simulink model "heli_master_2015b"  (R2015b)
settings: Solver=ode1  SolverMode=SingleTasking  StartTime=0.0  StopTime=inf  FixedStep=0.002  RelTol=1e-3
PostLoadFcn:
  | qc_set_target_type(getConfigSet(bdroot, 'QUARC Default Target Configuration'));
values from neighbouring files (symbols this model uses):
  K = P_predicted * C' * inv(C * P_predicted * C' + obj.W)    [ExtendedKalmanFilter.m]    (also in HighGainObserver.m = zeros(8, 2); StateFeedback.m = zeros(2, 6))
  lamb = block.ContStates.Data(3)    [BetterSimulation.m]    (also in FeedbackLinearization.m = x(3); dyn_ext_eps_meas.mat = [0 0 0 0 0 0 0 0 0 0 0 0 ... (30000 elements, 6000x5)]; e_-10_10_l_0_120_t_10.mat = [0 3.40359280049e-12 1.08295188827e-10 8.177826625e-10 3.426; e_-10_10_l_0_120_t_20.mat = [0 1.06295178385e-13 3.38915391498e-12 2.56636695446e-11 1.0)
  phi = block.ContStates.Data(1)    [BetterSimulation.m]    (also in FeedbackLinearization.m = x(1); dyn_ext_eps_meas.mat = [0 0 0 0 0 0 0 0 0 0 0 0 ... (18000 elements, 6000x3)]; e_-10_10_l_0_120_t_10.mat = [3.57789727367e-14 3.32260230971e-07 2.63920782562e-06 8.843; e_-10_10_l_0_120_t_20.mat = [3.52494450884e-15 1.04005854531e-08 8.29611824462e-08 2.791)
  R = diag(R_diag)    [compute_lqr_feedback.m]    (also in first_tvlqr_test.mat = [1  0; 0  1])
  vb = block.InputPort(2).Data    [BetterSimulation.m]    (also in analyze_eps_meas.m = [log_neg.signals(2).values; log_pos.signals(2).values]; dyn_ext_eps_meas.mat = [2.46662433384 2.46662437608 2.46662467016 2.46662546356 2.4; e_-10_10_l_0_120_t_10.mat = [3.03305943788 3.0306076999 3.02819113358 3.02581096907 3.02; e_-10_10_l_0_120_t_20.mat = [3.03305943788 3.0329822422 3.03290486178 3.03282733913 3.03)
  vf = block.InputPort(1).Data    [BetterSimulation.m]    (also in analyze_eps_meas.m = [log_neg.signals(1).values; log_pos.signals(1).values]; dyn_ext_eps_meas.mat = [2.46662433384 2.46662437608 2.46662467016 2.46662546356 2.4; e_-10_10_l_0_120_t_10.mat = [3.03305943788 3.03551133878 3.03792903521 3.04031223633 3.0; e_-10_10_l_0_120_t_20.mat = [3.03305943788 3.03313663866 3.03321405463 3.03329167331 3.0)
undefined symbols (not defined in the file or in its folder): HIL, qc_get_step_size
libraries: simulink_extras x25, quarc_library x4
(part 2 of 2)

== system heli_master_2015b/Feedback Controller/Trajectory Controller/Enabled Controller/Trajectory Controller Variants/TimeVariantLQR ==
  t : Inport
  x : Inport  Port=2
  t_d : Inport  Port=3
  phi_d : Inport  Port=4
  eps_d : Inport  Port=5
  lamb_d : Inport  Port=6
  vf_d : Inport  Port=7
  vb_d : Inport  Port=8
  MATLAB System : MATLABSystem  System=TimeVariantLQR  Q=Q  R=R  S=S  riccati_tau=riccati_tau  riccati_P_triu_tau=riccati_P_triu_tau  SimulateUsing=Code generation
      mask Type: TimeVariantLQR
      mask Display:
      | disp('TimeVariantLQR');
      | port_label('input',1,'Time');
      | port_label('input',2,'State');
      | port_label('input',3,'Traj Time');
      | port_label('input',4,'Traj Phi');
      | port_label('input',5,'Traj Eps');
      | port_label('input',6,'Traj Lamb');
      | port_label('input',7,'Traj Vf');
      | port_label('input',8,'Traj Vb');
      | port_label('output',1,'Control');
  TimeVariantLQR : Subsystem  Commented=on  mask(Time Variant LQR){Q_diag=[3, 50, 20, 2, 1, 5, 1, 1], R_diag=[1, 1], S_diag=[3, 50, 20, 2, 1, 5, 1, 1], riccati_step_width=0.1}
      mask help: LQR for LTV system resulting from linearization around desired trajectory.
      mask DialogControl Control2 Prompt: diag(Q):
      mask DialogControl Control3 Prompt: diag(R):
      mask DialogControl Control3_copy Prompt: diag(S):
      mask DialogControl Control4 Prompt: Riccati step width:
  u : Outport
  wires:
  MATLAB System/1 -> u/1
  vb_d/1 -> MATLAB System/8
  vf_d/1 -> MATLAB System/7
  lamb_d/1 -> MATLAB System/6
  eps_d/1 -> MATLAB System/5
  phi_d/1 -> MATLAB System/4
  t_d/1 -> MATLAB System/3
  x/1 -> MATLAB System/2
  t/1 -> MATLAB System/1

== system heli_master_2015b/Feedback Controller/Trajectory Controller/Enabled Controller/Trajectory Controller Variants/TimeVariantLQRI ==
  t : Inport
  x : Inport  Port=2
  t_d : Inport  Port=3
  phi_d : Inport  Port=4
  eps_d : Inport  Port=5
  lamb_d : Inport  Port=6
  vf_d : Inport  Port=7
  vb_d : Inport  Port=8
  MATLAB System : MATLABSystem  System=TimeVariantLQRI  Q=Q  R=R  S=S  riccati_tau=riccati_tau  riccati_P_triu_tau=riccati_P_triu_tau  step_width=0.002  SimulateUsing=Code generation
      mask Type: TimeVariantLQRI
      mask Display:
      | disp('TimeVariantLQRI');
      | port_label('input',1,'Time');
      | port_label('input',2,'State');
      | port_label('input',3,'Traj Time');
      | port_label('input',4,'Traj Phi');
      | port_label('input',5,'Traj Eps');
      | port_label('input',6,'Traj Lamb');
      | port_label('input',7,'Traj Vf');
      | port_label('input',8,'Traj Vb');
      | port_label('output',1,'Control');
      | port_label('output',2,'Debug');
  u : Outport
  wires:
  MATLAB System/1 -> u/1
  vb_d/1 -> MATLAB System/8
  vf_d/1 -> MATLAB System/7
  lamb_d/1 -> MATLAB System/6
  eps_d/1 -> MATLAB System/5
  phi_d/1 -> MATLAB System/4
  t_d/1 -> MATLAB System/3
  x/1 -> MATLAB System/2
  t/1 -> MATLAB System/1

== system heli_master_2015b/Feedback Controller/Trajectory Controller/Enabled Controller/Trajectory Controller Variants/Ad hoc PID/Conversion ==
  Vd [V] : Inport
  Vs [V] : Inport  Port=2
  Add : Sum
  Back gain : Gain  Gain=0.5
  Front gain : Gain  Gain=0.5
  Subtract : Sum  Inputs=+-
  Vf [V] : Outport
  Vb [V] : Outport  Port=2
  wires:
  Vd [V]/1 -> Subtract/2, Add/1
  Vs [V]/1 -> Subtract/1, Add/2
  Subtract/1 -> Back gain/1
  Back gain/1 -> Vb [V]/1
  Add/1 -> Front gain/1
  Front gain/1 -> Vf [V]/1

== system heli_master_2015b/Feedback Controller/Trajectory Controller/Enabled Controller/Trajectory Controller Variants/Ad hoc PID/Elevation controller ==
  e~ [rad] : Inport
  e~dot [rad/s] : Inport  Port=2
  e~c [rad] : Inport  Port=3
  Elevation controller : Subsystem
  Sum : Sum  Inputs=-+  SaturateOnIntegerOverflow=on  InputSameDT=on  OutDataTypeStr=Inherit: Same as first input
  V~s [V] : Outport  InitialOutput=0
  wires:
  Sum/1 -> Elevation controller/1(e~ [rad])
  Elevation controller/1(V~_s [V]) -> V~s [V]/1
  e~ [rad]/1 -> Sum/1
  e~dot [rad/s]/1 -> Elevation controller/2(e~_dot [rad/s])
  e~c [rad]/1 -> Sum/2

== system heli_master_2015b/Feedback Controller/Trajectory Controller/Enabled Controller/Trajectory Controller Variants/Ad hoc PID/Pitch controller ==
  p~c [rad] : Inport
  p~ [rad] : Inport  Port=2
  p~dot [rad/s] : Inport  Port=3
  Integrator : Integrator  LimitOutput=on
  Kd : Gain  Gain=3.5
  Ki : Gain  Gain=0.5
  Kp : Gain  Gain=8
  Saturation : Saturate  UpperLimit=10  LowerLimit=-10
  Sum : Sum  Inputs=+-
  Sum1 : Sum  Inputs=++-
  V~d [V] : Outport  InitialOutput=0
  wires:
  p~c [rad]/1 -> Sum/1
  p~ [rad]/1 -> Sum/2
  Sum/1 -> Ki/1, Kp/1
  p~dot [rad/s]/1 -> Kd/1
  Kp/1 -> Sum1/1
  Sum1/1 -> Saturation/1
  Saturation/1 -> V~d [V]/1
  Kd/1 -> Sum1/3
  Ki/1 -> Integrator/1
  Integrator/1 -> Sum1/2

== system heli_master_2015b/Feedback Controller/Trajectory Controller/Enabled Controller/Trajectory Controller Variants/Ad hoc PID/Travel controller ==
  lamb~c [rad] : Inport
  lamb~ [rad] : Inport  Port=2
  lamb~dot [rad/s] : Inport  Port=3
  Integrator : Integrator  LimitOutput=on  UpperSaturationLimit=45/180*pi  LowerSaturationLimit=-45/180*pi
  Kd : Gain  Gain=1.2
  Ki : Gain  Gain=0.02
  Kp : Gain  Gain=0.7
  Saturation : Saturate  UpperLimit=45/180*pi  LowerLimit=-45/180*pi
  Sum : Sum  Inputs=+-
  Sum1 : Sum  Inputs=++-
  p~c [rad] : Outport  InitialOutput=0
  wires:
  lamb~c [rad]/1 -> Sum/1
  lamb~ [rad]/1 -> Sum/2
  Sum/1 -> Ki/1, Kp/1
  lamb~dot [rad/s]/1 -> Kd/1
  Kp/1 -> Sum1/1
  Saturation/1 -> p~c [rad]/1
  Kd/1 -> Sum1/3
  Ki/1 -> Integrator/1
  Integrator/1 -> Sum1/2
  Sum1/1 -> Saturation/1

== system heli_master_2015b/Feedback Controller/Trajectory Controller/Enabled Controller/Trajectory Controller Variants/Joystick PID/Conversion ==
  Vd [V] : Inport
  Vs [V] : Inport  Port=2
  Add : Sum
  Back gain : Gain  Gain=0.5
  Front gain : Gain  Gain=0.5
  Subtract : Sum  Inputs=+-
  Vf [V] : Outport
  Vb [V] : Outport  Port=2
  wires:
  Vd [V]/1 -> Subtract/2, Add/1
  Vs [V]/1 -> Subtract/1, Add/2
  Subtract/1 -> Back gain/1
  Back gain/1 -> Vb [V]/1
  Add/1 -> Front gain/1
  Front gain/1 -> Vf [V]/1

== system heli_master_2015b/Feedback Controller/Trajectory Controller/Enabled Controller/Trajectory Controller Variants/Joystick PID/Elevation controller ==
  e~ [rad] : Inport
  e~dot [rad/s] : Inport  Port=2
  e~c [rad] : Inport  Port=3
  Elevation controller : Subsystem
  Sum : Sum  Inputs=-+  SaturateOnIntegerOverflow=on  InputSameDT=on  OutDataTypeStr=Inherit: Same as first input
  V~s [V] : Outport  InitialOutput=0
  wires:
  Sum/1 -> Elevation controller/1(e~ [rad])
  Elevation controller/1(V~_s [V]) -> V~s [V]/1
  e~ [rad]/1 -> Sum/1
  e~dot [rad/s]/1 -> Elevation controller/2(e~_dot [rad/s])
  e~c [rad]/1 -> Sum/2

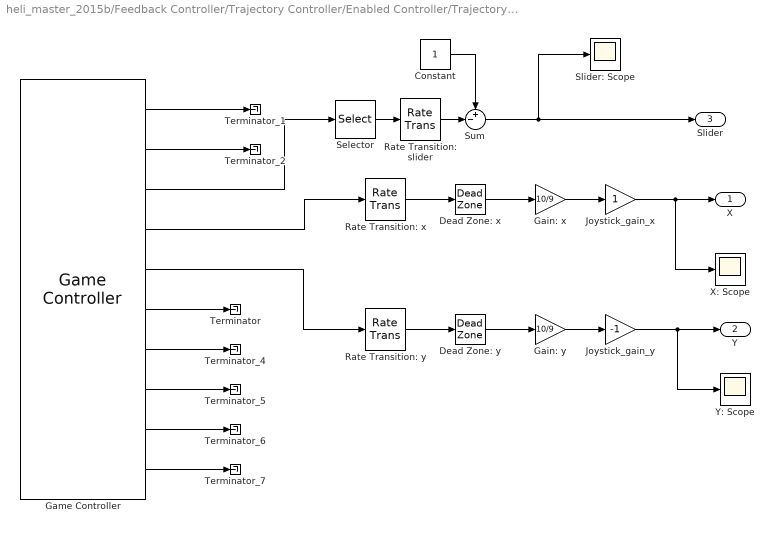
== system heli_master_2015b/Feedback Controller/Trajectory Controller/Enabled Controller/Trajectory Controller Variants/Joystick PID/Joystick ==
  Constant : Constant
  Dead Zone: x : DeadZone  LowerValue=-0.1  UpperValue=0.1  SaturateOnIntegerOverflow=on
  Dead Zone: y : DeadZone  LowerValue=-0.1  UpperValue=0.1  SaturateOnIntegerOverflow=on
  Gain: x : Gain  Gain=10/9
  Gain: y : Gain  Gain=10/9
  Game Controller : quarc_library/Devices/Peripherals/Target/Game Controller  controller=1  buffer_size=12  deadzone=[]  saturation=[]  sample_time=max(qc_get_step_size, 0.01)  auto_center=off  enabled=on
  Joystick_gain_x : Gain
  Joystick_gain_y : Gain  Gain=-1
  Rate Transition: slider : RateTransition
  Rate Transition: x : RateTransition
  Rate Transition: y : RateTransition
  Selector : Selector  InputPortWidth=2  IndexOptions=Index vector (dialog)  Indices=1  OutputSizes=1
  Slider: Scope : Scope
  Sum : Sum  Inputs=+-|
  Terminator : Terminator
  Terminator_{1..2,4..7} (6 alike) : Terminator
  X: Scope : Scope
  Y: Scope : Scope
  X : Outport
  Y : Outport  Port=2
  Slider : Outport  Port=3
  wires:
  Rate Transition: y/1 -> Dead Zone: y/1
  Rate Transition: x/1 -> Dead Zone: x/1
  Game Controller/5 -> Rate Transition: y/1
  Game Controller/4 -> Rate Transition: x/1
  Game Controller/1 -> Terminator_1/1
  Game Controller/2 -> Terminator_2/1
  Game Controller/7 -> Terminator_4/1
  Game Controller/8 -> Terminator_5/1
  Game Controller/9 -> Terminator_6/1
  Game Controller/10 -> Terminator_7/1
  Game Controller/3 -> Selector/1
  Game Controller/6 -> Terminator/1
  Dead Zone: x/1 -> Gain: x/1
  Dead Zone: y/1 -> Gain: y/1
  Gain: x/1 -> Joystick_gain_x/1
  Gain: y/1 -> Joystick_gain_y/1
  Joystick_gain_x/1 -> X/1, X: Scope/1
  Joystick_gain_y/1 -> Y: Scope/1, Y/1
  Sum/1 -> Slider/1, Slider: Scope/1
  Constant/1 -> Sum/1
  Selector/1 -> Rate Transition: slider/1
  Rate Transition: slider/1 -> Sum/2

== system heli_master_2015b/Feedback Controller/Trajectory Controller/Enabled Controller/Trajectory Controller Variants/Joystick PID/Pitch controller ==
  p~c [rad] : Inport
  p~ [rad] : Inport  Port=2
  p~dot [rad/s] : Inport  Port=3
  Integrator : Integrator  LimitOutput=on
  Kd : Gain  Gain=3.5
  Ki : Gain  Gain=0.5
  Kp : Gain  Gain=8
  Saturation : Saturate  UpperLimit=10  LowerLimit=-10
  Sum : Sum  Inputs=+-
  Sum1 : Sum  Inputs=++-
  V~d [V] : Outport  InitialOutput=0
  wires:
  p~c [rad]/1 -> Sum/1
  p~ [rad]/1 -> Sum/2
  Sum/1 -> Ki/1, Kp/1
  p~dot [rad/s]/1 -> Kd/1
  Kp/1 -> Sum1/1
  Sum1/1 -> Saturation/1
  Saturation/1 -> V~d [V]/1
  Kd/1 -> Sum1/3
  Ki/1 -> Integrator/1
  Integrator/1 -> Sum1/2

== system heli_master_2015b/Feedback Controller/Trajectory Controller/Enabled Controller/Trajectory Controller Variants/Joystick PID/Travel controller ==
  lamb~c [rad] : Inport
  lamb~ [rad] : Inport  Port=2
  lamb~dot [rad/s] : Inport  Port=3
  Integrator : Integrator  LimitOutput=on
  Kd : Gain  Gain=1.8
  Ki : Gain  Gain=0.005
  Kp : Gain  Gain=1.5
  Saturation : Saturate  UpperLimit=20  LowerLimit=-20
  Sum : Sum  Inputs=+-
  Sum1 : Sum  Inputs=++-
  p~c [rad] : Outport  InitialOutput=0
  wires:
  lamb~c [rad]/1 -> Sum/1
  lamb~ [rad]/1 -> Sum/2
  Sum/1 -> Ki/1, Kp/1
  lamb~dot [rad/s]/1 -> Kd/1
  Kp/1 -> Sum1/1
  Saturation/1 -> p~c [rad]/1
  Kd/1 -> Sum1/3
  Ki/1 -> Integrator/1
  Integrator/1 -> Sum1/2
  Sum1/1 -> Saturation/1

== system heli_master_2015b/Feedback Controller/Trajectory Controller/Enabled Controller/Trajectory Controller Variants/TimeVariantLQR/TimeVariantLQR ==
  t : Inport
  x : Inport  Port=2
  t_d : Inport  Port=3
  phi_d : Inport  Port=4
  eps_d : Inport  Port=5
  lamb_d : Inport  Port=6
  vf_d : Inport  Port=7
  vb_d : Inport  Port=8
  Constant : Constant  Value=Q_diag
  Constant1 : Constant  Value=R_diag
  Constant2 : Constant  Value=S_diag
  Constant3 : Constant  Value=riccati_step_width
  MATLAB Function : MATLAB Function  TreatAsAtomicUnit=on
  u : Outport
  wires:
  MATLAB Function/1(u) -> u/1
  x/1 -> MATLAB Function/2(x)
  t/1 -> MATLAB Function/1(t)
  t_d/1 -> MATLAB Function/3(t_d)
  phi_d/1 -> MATLAB Function/4(phi_d)
  eps_d/1 -> MATLAB Function/5(eps_d)
  lamb_d/1 -> MATLAB Function/6(lamb_d)
  vf_d/1 -> MATLAB Function/7(vf_d)
  vb_d/1 -> MATLAB Function/8(vb_d)
  Constant/1 -> MATLAB Function/9(Q_diag)
  Constant1/1 -> MATLAB Function/10(R_diag)
  Constant2/1 -> MATLAB Function/11(S_diag)
  Constant3/1 -> MATLAB Function/12(riccati_step_width)

== system heli_master_2015b/Feedback Controller/Trajectory Controller/Enabled Controller/Trajectory Controller Variants/Ad hoc PID/Elevation controller/Elevation controller ==
  e~ [rad] : Inport
  e~_dot [rad/s] : Inport  Port=2
  Integrator : Integrator  LimitOutput=on
  K_ed : Gain  Gain=20  SaturateOnIntegerOverflow=on  OutDataTypeStr=Inherit: Same as input  ParamDataTypeStr=Inherit: Same as input
  K_ei : Gain  Gain=20  SaturateOnIntegerOverflow=on  OutDataTypeStr=Inherit: Same as input  ParamDataTypeStr=Inherit: Same as input
  K_ep : Gain  Gain=30  SaturateOnIntegerOverflow=on  OutDataTypeStr=Inherit: Same as input  ParamDataTypeStr=Inherit: Same as input
  Sum : Sum  Inputs=++-  SaturateOnIntegerOverflow=on  InputSameDT=on  OutDataTypeStr=Inherit: Same as first input
  V~_s [V] : Outport  InitialOutput=0
  wires:
  K_ei/1 -> Integrator/1
  Integrator/1 -> Sum/1
  Sum/1 -> V~_s [V]/1
  e~_dot [rad/s]/1 -> K_ed/1
  K_ed/1 -> Sum/3
  K_ep/1 -> Sum/2
  e~ [rad]/1 -> K_ep/1, K_ei/1

== system heli_master_2015b/Feedback Controller/Trajectory Controller/Enabled Controller/Trajectory Controller Variants/Joystick PID/Elevation controller/Elevation controller ==
  e~ [rad] : Inport
  e~_dot [rad/s] : Inport  Port=2
  Integrator : Integrator  LimitOutput=on
  K_ed : Gain  Gain=12  SaturateOnIntegerOverflow=on  OutDataTypeStr=Inherit: Same as input  ParamDataTypeStr=Inherit: Same as input
  K_ei : Gain  Gain=5  SaturateOnIntegerOverflow=on  OutDataTypeStr=Inherit: Same as input  ParamDataTypeStr=Inherit: Same as input
  K_ep : Gain  Gain=15  SaturateOnIntegerOverflow=on  OutDataTypeStr=Inherit: Same as input  ParamDataTypeStr=Inherit: Same as input
  Sum : Sum  Inputs=++-  SaturateOnIntegerOverflow=on  InputSameDT=on  OutDataTypeStr=Inherit: Same as first input
  V~_s [V] : Outport  InitialOutput=0
  wires:
  K_ei/1 -> Integrator/1
  Integrator/1 -> Sum/1
  Sum/1 -> V~_s [V]/1
  e~_dot [rad/s]/1 -> K_ed/1
  K_ed/1 -> Sum/3
  K_ep/1 -> Sum/2
  e~ [rad]/1 -> K_ep/1, K_ei/1

== matlab function heli_master_2015b/Feedback Controller/Trajectory Controller/Enabled Controller/Evaluate Trajectory ==
  data: traj_t input; traj_phi input; traj_eps input; traj_lamb input; traj_vf input; traj_vb input; vals output; t input
function vals  = fcn(traj_t, traj_phi, traj_eps, traj_lamb, traj_vf, traj_vb, t)
traj = struct('t', traj_t, 'phi', traj_phi, 'eps', traj_eps, 'lamb', traj_lamb, 'vf', traj_vf, 'vb', traj_vb);
traj_eval = eval_trajectory(traj, t);

vals = zeros(5, 1);
vals(1) = traj_eval.vf(1);
vals(2) = traj_eval.vb(1);
vals(3) = traj_eval.phi(1);
vals(4) = traj_eval.eps(1);
vals(5) = traj_eval.lamb(1);

== matlab function heli_master_2015b/Feedback Controller/Enable Ramping Controller ==
  data: start_stop_trajectory input; enable_ramping output; trajectory_ts input; time input; auto_switch_off input
function enable_ramping = fcn(start_stop_trajectory, trajectory_ts, time, auto_switch_off)
persistent last_start_stop_trajectory trajectory_t0 running_trajectory

if isempty(last_start_stop_trajectory)
    last_start_stop_trajectory = 1;
    trajectory_t0 = time;
    running_trajectory = 0;
end

if start_stop_trajectory == 1 && last_start_stop_trajectory ~= 1
    running_trajectory = 1;
    trajectory_t0 = time;
end
if start_stop_trajectory == -1 && last_start_stop_trajectory ~= -1
    running_trajectory = 0;
end
last_start_stop_trajectory = start_stop_trajectory;

trajectory_length = trajectory_ts(end);

if time - trajectory_t0 > trajectory_length && auto_switch_off
    running_trajectory = 0;
end


if running_trajectory
    enable_ramping = -1;
else
    enable_ramping = 1;
end

== matlab function heli_master_2015b/Feedback Controller/Trajectory Controller/Enabled Controller/Trajectory Controller Variants/TimeVariantLQR/TimeVariantLQR/MATLAB Function ==
  data: t input; u output; x input; t_d input; phi_d input; eps_d input; lamb_d input; vf_d input; vb_d input; Q_diag input; R_diag input; S_diag input; riccati_step_width input
function u = fcn(t, x, t_d, phi_d, eps_d, lamb_d, vf_d, vb_d, Q_diag, R_diag, S_diag, riccati_step_width)
persistent sys

if isempty(sys)
    sys = TimeVariantLQR();
    
    sys.Q_diag = Q_diag;
    sys.R_diag = R_diag;
    sys.S_diag = S_diag;
    sys.riccati_step_width = riccati_step_width;
    
    sys.setup(t, x, t_d, phi_d, eps_d, lamb_d, vf_d, vb_d)
end

u = sys.step(t, x, t_d, phi_d, eps_d, lamb_d, vf_d, vb_d);

== matlab function heli_master_2015b/Observer/EKF/Estimator/MATLAB Function ==
  data: y input; u input; x output; x0 input; P_diag input; N_diag input; W_diag input; step_width input
function x = fcn(y, u, x0, P_diag, N_diag, W_diag, step_width)
persistent sys

if isempty(sys)
    sys = ExtendedKalmanFilter();
    sys.x0 = x0;
    sys.P_diag = P_diag;
    sys.N_diag = N_diag;
    sys.W_diag = W_diag;
    sys.step_width = step_width;
    
    sys.setup(y, u)
    sys.reset()
end

x = sys.step(y, u);

== matlab function heli_master_2015b/Observer/Enable EKF ==
  data: x_ekf input; ekf_enabled output; x_filter input; time input; divergence output
function [ekf_enabled, divergence]= fcn(x_ekf, x_filter, time)
persistent last_threshold_violation

if isempty(last_threshold_violation)
    last_threshold_violation = time;
end

angle_diff_deg_rms_threshold = 2;
violation_timeout = 5;

angle_diff_deg_rms = rms([x_ekf(1) + x_ekf(9) - x_filter(1) - x_filter(9); x_ekf(2:3) - x_filter(2:3)]) / pi * 180;

if angle_diff_deg_rms > angle_diff_deg_rms_threshold && x_filter(2) < -25 / 180 * pi
    last_threshold_violation = time;
end

if time - last_threshold_violation > violation_timeout
    ekf_enabled = 1;
else
    ekf_enabled = -1;
end

divergence = angle_diff_deg_rms;
